simulink model "intro_sim_b"  (R2021b)
settings: Solver=VariableStepAuto  StartTime=0.0  StopTime=10.0  RelTol=1e-3
settings Model: Creator=Juho  LastModifiedBy=Juho

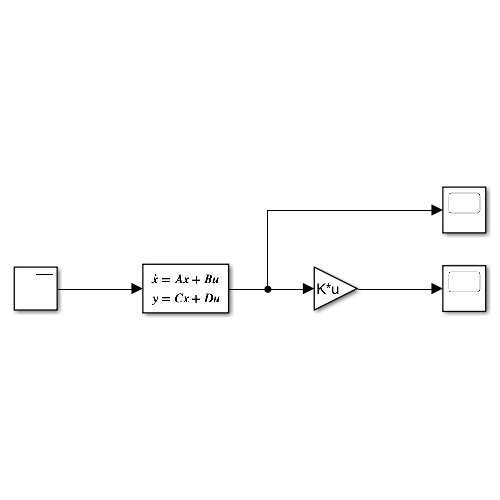
[thumbnail: Simulink's stored preview of the top-level diagram]
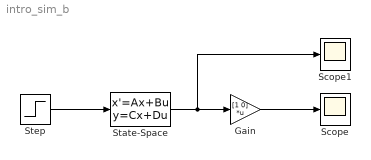
== system intro_sim_b ==
  Gain : Gain  Gain=[1 0]  Multiplication=Matrix(K*u)
  Scope : Scope
  Scope1 : Scope
  State-Space : StateSpace  A=[0 1; -4 -2]  B=[0; 4]  C=eye(2)  D=zeros(2, 1)  InitialCondition=0
  Step : Step  Time=0  SampleTime=0
  wires:
  Step/1 -> State-Space/1
  Gain/1 -> Scope/1
  State-Space/1 -> Gain/1, Scope1/1
